simulink model "performancemetricsmclab"  (R2017a)
settings: Solver=FixedStepAuto  StartTime=0.0  StopTime=simtime  FixedStep=0.01  RelTol=1e-3
settings Model: Creator=ONLyn  LastModifiedBy=torees

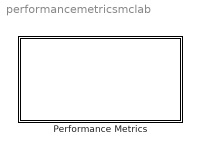
== system performancemetricsmclab ==
  "Performance Metrics " : Subsystem

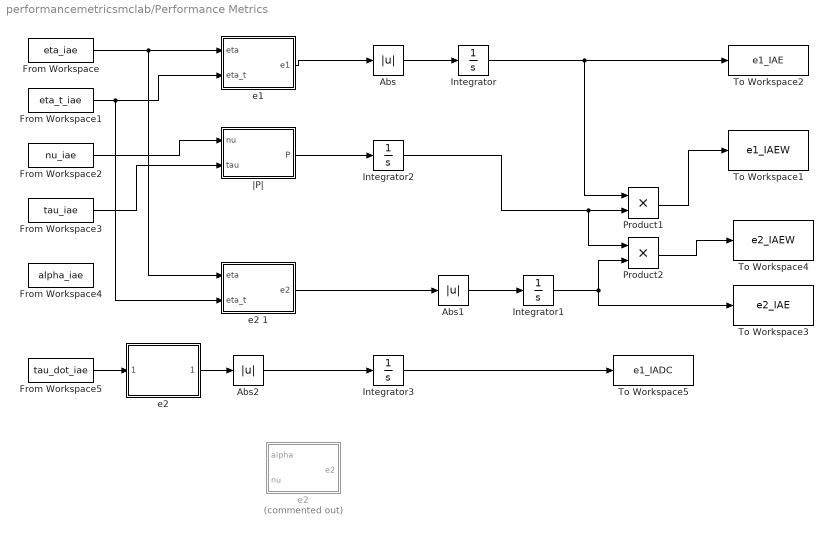
== system performancemetricsmclab/Performance Metrics  ==
  Abs : Abs
  Abs1 : Abs
  Abs2 : Abs
  From Workspace : FromWorkspace  VariableName=eta_iae  SampleTime=0
  From Workspace1 : FromWorkspace  VariableName=eta_t_iae  SampleTime=0
  From Workspace2 : FromWorkspace  VariableName=nu_iae  SampleTime=0
  From Workspace3 : FromWorkspace  VariableName=tau_iae  SampleTime=0
  From Workspace4 : FromWorkspace  VariableName=alpha_iae  SampleTime=0
  From Workspace5 : FromWorkspace  VariableName=tau_dot_iae  SampleTime=0
  Integrator{,1..3} (4 alike) : Integrator
  Product1 : Product
  Product2 : Product
  To Workspace1 : ToWorkspace  VariableName=e1_IAEW  SampleTime=-1
  To Workspace2 : ToWorkspace  VariableName=e1_IAE  SampleTime=-1
  To Workspace3 : ToWorkspace  VariableName=e2_IAE  SampleTime=-1
  To Workspace4 : ToWorkspace  VariableName=e2_IAEW  SampleTime=-1
  To Workspace5 : ToWorkspace  VariableName=e1_IADC  SampleTime=-1
  e1 : MATLAB Function  TreatAsAtomicUnit=on
  e2 : MATLAB Function  TreatAsAtomicUnit=on
  "e2 " : MATLAB Function  Commented=on  TreatAsAtomicUnit=on
  e2 1 : MATLAB Function  TreatAsAtomicUnit=on
  |P| : MATLAB Function  TreatAsAtomicUnit=on
  wires:
  Integrator/1 -> Product1/1, To Workspace2/1
  e1/1(e1) -> Abs/1
  Abs/1 -> Integrator/1
  |P|/1(P) -> Integrator2/1
  Integrator2/1 -> Product2/1, Product1/2
  Product1/1 -> To Workspace1/1
  From Workspace/1 -> e2 1/1(eta), e1/1(eta)
  From Workspace2/1 -> |P|/1(nu)
  e2 1/1(e2) -> Abs1/1
  Abs1/1 -> Integrator1/1
  Integrator1/1 -> Product2/2, To Workspace3/1
  Product2/1 -> To Workspace4/1
  From Workspace1/1 -> e2 1/2(eta_t), e1/2(eta_t)
  From Workspace3/1 -> |P|/2(tau)
  From Workspace5/1 -> e2/1(tau_dot_in)
  Abs2/1 -> Integrator3/1
  Integrator3/1 -> To Workspace5/1
  e2/1(tau_dot) -> Abs2/1

== matlab function performancemetricsmclab/Performance Metrics /e2 ==
  data: tau_dot output; tau_dot_in input
function tau_dot = fcn(tau_dot_in)

tau1 = tau_dot_in(1);
tau2 = tau_dot_in(2);
tau3 = tau_dot_in(3);



tau_dot = sqrt((tau1^2) + (tau2^2) + (tau3^2));

== matlab function performancemetricsmclab/Performance Metrics /e2 1 ==
  data: eta input; eta_t input; e2 output
function e2 = fcn(eta,eta_t )

x = eta(1);
x_d = eta_t(1);
y=eta(2);
y_d=eta_t(2);
psi=eta(3);
e2=abs(-sin(psi)*(x-x_d)+cos(psi)*(y-y_d));
end

== matlab function performancemetricsmclab/Performance Metrics /e1 ==
  data: e1 output; eta input; eta_t input
function e1 = fcn(eta,eta_t)

x = eta(1);
y = eta(2);
psi = eta(3);

x_t = eta_t(1);
y_t = eta_t(2);
psi_t = eta_t(3);

x_tilde = x-x_t;
y_tilde = y-y_t;
psi_tilde = psi-psi_t;

e1 = sqrt((x_tilde^2)/4 + (y_tilde^2)/4 + (psi_tilde^2)/(pi/2));

== matlab function performancemetricsmclab/Performance Metrics /e2  ==
  data: alpha input; nu input; e2 output
function e2 = fcn(alpha,nu )

u = nu(1);
v = nu(2);
r = nu(3);
% u_norm = abs(u)/0.4754;
% v_norm = abs(v)/0.1367; %max speeds
% r_norm = abs(r)/0.08951;

u_t = alpha(1);
v_t = alpha(2);
r_t = alpha(3);
% u_t_norm = abs(u_t)/0.4754;
% v_t_norm = abs(v_t)/0.1367; %max speeds
% r_t_norm = abs(r_t)/0.08951;

% u_tilde = u_norm-u_t_norm;
% v_tilde = v_norm-v_t_norm;
% r_tilde = r_norm-r_t_norm;
u_tilde = u - u_t;
v_tilde = v - v_t;
r_tilde = r - r_t;

e2 = sqrt(u_tilde^2 + v_tilde^2 + r_tilde^2);
end

== matlab function performancemetricsmclab/Performance Metrics /|P| ==
  data: nu input; P output; tau input
function P  = fcn(nu, tau)
P = abs(nu'*tau);
